simulink model "ArduinoHub"  (R2019b)
settings: Solver=FixedStepDiscrete  StartTime=0.0  StopTime=inf  FixedStep=1  RelTol=1e-3
libraries: arduinolib x2
settings Model: SILPILModeSetting=veronly  ExtModeTrigDuration=2  Creator=wuyuanyi  LastModifiedBy=wuyuanyi
settings OptimizationCC: DefaultParameterBehavior=Inlined  StrengthReduction=on  PassReuseOutputArgsAs=Individual arguments  ZeroExternalMemoryAtStartup=off  ZeroInternalMemoryAtStartup=off  MaxStackSize=64  OptimizeBlockOrder=speed  OptimizationPriority=Speed  OptimizationCustomize=off  MultiThreadedLoops=on  EfficientTunableParamExpr=on
settings DebuggingCC: ParameterTunabilityLossMsg=error
settings HardwareCC: ProdBitPerInt=16  ProdBitPerPointer=16  ProdBitPerSizeT=16  ProdBitPerPtrDiffT=16  ProdLargestAtomicFloat=Double  ProdWordSize=8  ProdLongLongMode=on  ProdHWDeviceType=Atmel->AVR
settings SFSimCC: MATLABDynamicMemAlloc=off  CustomCodeUndefinedFunction=UseInterfaceOnly
settings RTWCC: SystemTargetFile=ert.tlc  HardwareBoard=Arduino Uno  TLCOptions=-aInlineSetEventsForThisBaseRateFcn=TLC_FALSE -aSuppressMultiTaskScheduler=TLC_FALSE -aRateBasedStepFcn=1  TemplateMakefile=ert_default_tmf  GenerateReport=on  Toolchain=Arduino AVR  BuildConfiguration=Faster Runs  IncludeHyperlinkInReport=on  LaunchReport=on  GenerateTraceInfo=on  GenerateTraceReport=on  GenerateTraceReportSl=on  GenerateTraceReportSf=on  GenerateTraceReportEml=on
settings CodeAppCC: ForceParamTrailComments=on  IgnoreCustomStorageClasses=off  OperatorAnnotations=on  SimulinkDataObjDesc=on  SFDataObjDesc=on  InsertBlockDesc=on
settings ERTTargetCC: TargetLangStandard=C99 (ISO)  SupportAbsoluteTime=off  SupportNonFinite=off  SupportComplex=off  ExtModeStaticAllocSize=250  RootIOFormat=Structure reference

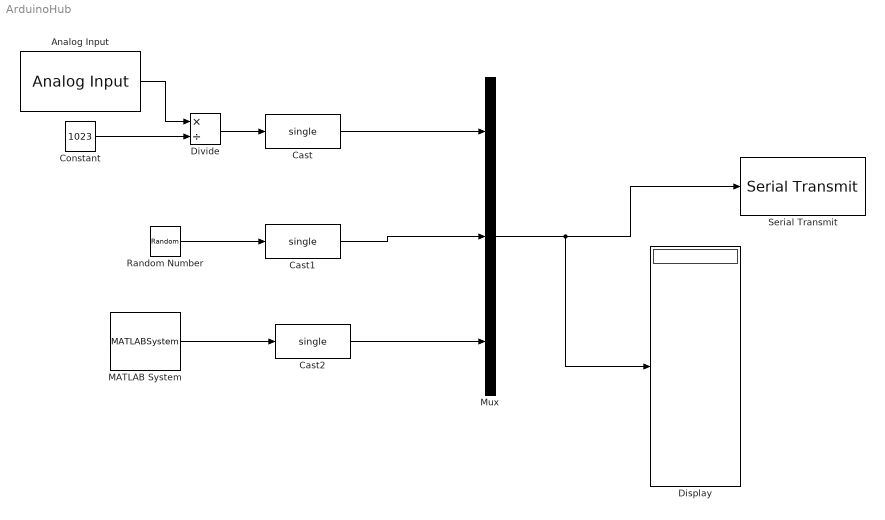
== system ArduinoHub ==
  Analog Input : arduinolib/Analog Input  pinNumber=4  ReadResultsOnly=off  ConversionTriggerSource=Software  ExternalTriggerType=uint32(0)  OutputDataType=uint16  EnableConversionCompleteNotify=off  EnableOuputStatus=off  SampleTime=1  blockPlatform=arduino
  Cast : DataTypeConversion  OutDataTypeStr=single
  Cast1 : DataTypeConversion  OutDataTypeStr=single  LockScale=on
  Cast2 : DataTypeConversion  OutDataTypeStr=single
  Constant : Constant  Value=1023
  Display : Display
  Divide : Product  Inputs=*/
  MATLAB System : MATLABSystem  System=DS18B20  port=7  SampleTime=1
      mask Type: DS18B20
      mask Display:
      | disp('DS18B20');
      | port_label('output',1,'y');
  Mux : Mux  Inputs=3
  Random Number : RandomNumber  SampleTime=1
  Serial Transmit : arduinolib/Serial Transmit  portNumber=0  sendmode=write  sendformat=Decimal  floatprecision=2  blockPlatform=arduino
      settings: SourceProductName=Simulink Support Package for Arduino Hardware
  wires:
  Mux/1 -> Display/1, Serial Transmit/1
  Analog Input/1 -> Divide/1
  Divide/1 -> Cast/1
  Cast/1 -> Mux/1
  Constant/1 -> Divide/2
  Cast1/1 -> Mux/2
  Random Number/1 -> Cast1/1
  MATLAB System/1 -> Cast2/1
  Cast2/1 -> Mux/3
